simulink model "EJ_01_c"  (R2018a)
settings: Solver=ode23t  StartTime=0.0  StopTime=7  FixedStep=0.01  MaxStep=0.05  RelTol=1e-3  EnableMultiTasking=on
PreLoadFcn:
  | mdl_puma560
values from neighbouring files (symbols this model uses):
  messi = RobotInit(pert)    [Ej_01.m]
  q0 = [0 -pi/2]    [Ej_01.m]
undefined symbols (not defined in the file or in its folder): slcoulomb
libraries: roblocks x6, simulink x1
settings Model: ExtModeTrigMode=oneshot  ExtModeArmWhenConnect=off  Creator=pic  LastModifiedBy=sebas
settings SolverCC: ZeroCrossControl=DisableAll
settings DataIOCC: SaveFormat=Array  SignalLoggingSaveFormat=ModelDataLogs  ReturnWorkspaceOutputs=on  TimeSaveName=t  OutputSaveName=y  ReturnWorkspaceOutputsName=ctorque
settings OptimizationCC: BlockReduction=off  BooleanDataType=off  ExpressionDepthLimit=2147483647  InitFltsAndDblsToZero=on  LifeSpan=inf
settings DebuggingCC: SaveWithParameterizedLinksMsg=none  UnderspecifiedInitializationDetection=Classic  MergeDetectMultiDrivingBlocksExec=none  SignalResolutionControl=TryResolveAllWithWarning  MultiTaskDSMMsg=warning  MultiTaskCondExecSysMsg=none  FcnCallInpInsideContextMsg=warning  AllowSymbolicDim=off  StateNameClashWarn=warning  SFUnexpectedBacktrackingDiag=warning  SFNoUnconditionalDefaultTransitionDiag=warning  SFExecutionAtInitializationDiag=none
settings HardwareCC: ProdBitPerPointer=32  ProdBitPerSizeT=32  ProdBitPerPtrDiffT=32  ProdLargestAtomicFloat=None  ProdIntDivRoundTo=Undefined  ProdEndianess=Unspecified  ProdWordSize=32  ProdHWDeviceType=32-bit Generic  TargetUnknown=on
settings ModelReferenceCC: PropagateSignalLabelsOutOfModel=off
settings CodeAppCC: StateflowObjectComments=on
settings GRTTargetCC: TargetLangStandard=C89/C90 (ANSI)  ModelReferenceCompliant=off  CompOptLevelCompliant=off  GeneratePreprocessorConditionals=Disable all  CombineOutputUpdateFcns=off  MatFileLogging=off  GRTInterface=on
settings ConfigComp: CovMetricSettings=dw  CovHtmlReporting=on  CovSaveCumulativeToWorkspaceVar=on  CovSaveSingleToWorkspaceVar=on  CovExternalEMLEnable=off

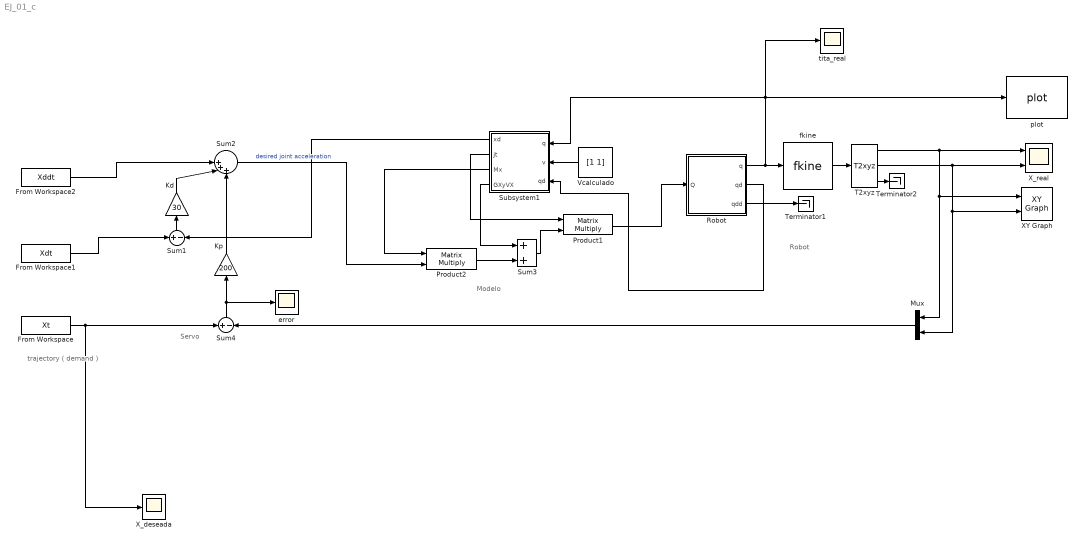
== system EJ_01_c ==
  note: Modelo
  note: trajectory
      | ( demand )
  note: Servo
  note: Robot
  From Workspace : FromWorkspace  VariableName=Xt  OutputAfterFinalValue=Holding final value
  From Workspace1 : FromWorkspace  VariableName=Xdt  OutputAfterFinalValue=Holding final value
  From Workspace2 : FromWorkspace  VariableName=Xddt  OutputAfterFinalValue=Holding final value
  Kd : Gain  Gain=30  SaturateOnIntegerOverflow=on  OutDataTypeStr=Inherit: Same as input  ParamDataTypeStr=Inherit: Same as input
  Kp : Gain  Gain=200  SaturateOnIntegerOverflow=on  OutDataTypeStr=Inherit: Same as input  ParamDataTypeStr=Inherit: Same as input
  Mux : Mux  Inputs=2
  Product1 : Product  Multiplication=Matrix(*)
  Product2 : Product  Multiplication=Matrix(*)
  Robot : Subsystem  AncestorBlock=roblocks/Arm/Robot  mask{robot=messi, q0=q0}
      mask prompts: robot "Robot object"; q0 "Initial state"
      mask help: Rigid-body dynamic model of robot.
      mask init:
      | if isa(robot, 'SerialLink')
      |     rname = robot.name;
      |     %fprintf('**robot name is %s\n', rname);
      | else
      |     rname = '';
      |     n = 0
      | end
      mask Help:
      | Simulates the forward (direct) rigid-body dynamics of the robot described
      | by the given robot object.  For given applied joint torque/force it computes
      | the instaneous joint coordinates, velocities and acclerations.
      | 
      | 
      | <b>Parameters::</b>
      | 
      | robot (SerialLink) a dynamic model of an N-link serial link manipulator
      | q0 (1xN)  Initial joint coordinates
      | 
      | <b>Inputs::</b>
      | 
      | Q (1xN) the generalized joint force (torque or force) required to achieve
      | the motion state (q, qd, qdd).
      | 
      | <b>Outputs::</b>
      | 
      | q (1xN) joint coordinates
      | qd (1xN) joint coordinate velocity
      | qdd (1xN) joint coordinate acceleration
      | 
      | 
      | <b>Notes::</b>
      | 
      | - Required to simulate robot rigid body motion.
      | - Implemented using the recursive Newton-Euler scheme (RNE).
      | - A wrapper for the Toolbox method accel() which in turn depends on the
      |   method rne().
      mask Display:
      | port_label('input', 1, 'Q')
      | port_label('output', 1, 'q')
      | port_label('output', 2, 'qd')
      | port_label('output', 3, 'qdd')
      | text(0.1, 0.9,  rname, 'horizontalAlignment', 'left')
  Subsystem1 : Subsystem
  Sum1 : Sum  Inputs=+|-  SaturateOnIntegerOverflow=on  InputSameDT=on  OutDataTypeStr=Inherit: Same as first input
  Sum2 : Sum  Inputs=||+++  SaturateOnIntegerOverflow=on  InputSameDT=on  OutDataTypeStr=Inherit: Same as first input
  Sum3 : Sum
  Sum4 : Sum  Inputs=+|-  SaturateOnIntegerOverflow=on  InputSameDT=on  OutDataTypeStr=Inherit: Same as first input
  T2xyz : roblocks/Toolbox/T2xyz
  Terminator1 : Terminator
  Terminator2 : Terminator
  Vcalculado : Constant  Value=[1 1]
  XY Graph : simulink/Sinks/XY Graph  xmin=0  xmax=2  ymin=-1.5  ymax=2  st=-1
  X_deseada : Scope
  X_real : Scope  NumInputPorts=2
  error : Scope
  fkine : roblocks/Arm/fkine  robot=messi
  plot : roblocks/Arm/plot  robot=messi  fps=10  holdplot=on
  tita_real : Scope
  wires:
  Robot/3(qdd) -> Terminator1/1
  fkine/1 -> T2xyz/1
  T2xyz/2 -> Mux/2, XY Graph/2, X_real/2
  T2xyz/1 -> Mux/1, XY Graph/1, X_real/1
  Sum1/1 -> Kd/1
  Sum4/1 -> Kp/1, error/1
  From Workspace/1 -> Sum4/1, X_deseada/1
  From Workspace1/1 -> Sum1/1
  Kp/1 -> Sum2/3
  Kd/1 -> Sum2/2
  From Workspace2/1 -> Sum2/1
  Mux/1 -> Sum4/2
  Robot/1(q) -> tita_real/1, Subsystem1/1(q), plot/1, fkine/1
  Robot/2(qd) -> Subsystem1/3(qd)
  T2xyz/3 -> Terminator2/1
  Vcalculado/1 -> Subsystem1/2(v)
  Product1/1 -> Robot/1(Q)
  Subsystem1/1("xd ") -> Sum1/2
  Subsystem1/3(Mx) -> Product2/1
  Sum2/1 -> Product2/2  "desired joint acceleration"
  Subsystem1/2(jt) -> Product1/1
  Sum3/1 -> Product1/2
  Subsystem1/4(GXyVX) -> Sum3/1
  Product2/1 -> Sum3/2

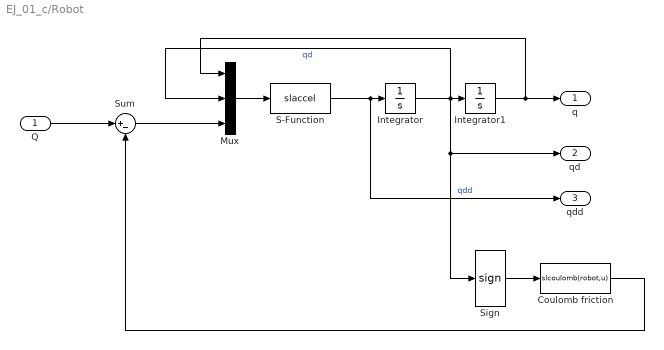
== system EJ_01_c/Robot ==
  Q : Inport
  Coulomb friction : MATLABFcn  MATLABFcn=slcoulomb(robot,u)  OutputDimensions=[robot.n 1]  Output1D=off
  Integrator : Integrator
  Integrator1 : Integrator  InitialCondition=q0
  Mux : Mux  Inputs=3
  S-Function : S-Function  FunctionName=slaccel  Parameters=robot  SFunctionDeploymentMode=off  EnableBusSupport=off
  Sign : Signum
  Sum : Sum  Inputs=|+-
  q : Outport
  qd : Outport  Port=2
  qdd : Outport  Port=3
  wires:
  S-Function/1 -> qdd/1, Integrator/1  "qdd"
  Mux/1 -> S-Function/1
  Integrator/1 -> Sign/1, qd/1, Integrator1/1, Mux/2  "qd"
  Integrator1/1 -> q/1, Mux/1
  Q/1 -> Sum/1
  Sum/1 -> Mux/3
  Coulomb friction/1 -> Sum/2
  Sign/1 -> Coulomb friction/1

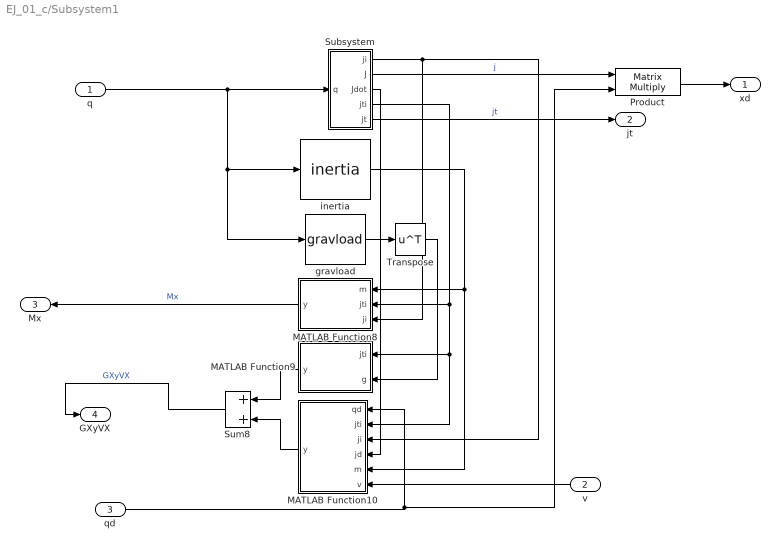
== system EJ_01_c/Subsystem1 ==
  q : Inport
  v : Inport  Port=2
  qd : Inport  Port=3
  MATLAB Function10 : MATLAB Function  TreatAsAtomicUnit=on
  MATLAB Function8 : MATLAB Function  TreatAsAtomicUnit=on
  MATLAB Function9 : MATLAB Function  TreatAsAtomicUnit=on
  Product : Product  Multiplication=Matrix(*)
  Subsystem : Subsystem
  Sum8 : Sum
  Transpose : Math  Operator=transpose  SaturateOnIntegerOverflow=on
  gravload : roblocks/Arm/gravload  robot=messi
  inertia : roblocks/Arm/inertia  robot=messi
  "xd " : Outport  VectorParamsAs1DForOutWhenUnconnected=on
  jt : Outport  Port=2  VectorParamsAs1DForOutWhenUnconnected=on
  Mx : Outport  Port=3  VectorParamsAs1DForOutWhenUnconnected=on
  GXyVX : Outport  Port=4  VectorParamsAs1DForOutWhenUnconnected=on
  wires:
  Subsystem/1(ji) -> MATLAB Function8/3(ji), MATLAB Function10/3(ji)
  q/1 -> gravload/1, inertia/1, Subsystem/1(q)
  Subsystem/4(jti) -> MATLAB Function8/2(jti), MATLAB Function9/1(jti), MATLAB Function10/2(jti)
  MATLAB Function9/1(y) -> Sum8/1
  Sum8/1 -> GXyVX/1  "GXyVX"
  Subsystem/3(Jdot) -> MATLAB Function10/4(jd)
  MATLAB Function10/1(y) -> Sum8/2
  inertia/1 -> MATLAB Function8/1(m), MATLAB Function10/5(m)
  Subsystem/5(jt) -> jt/1  "jt"
  v/1 -> MATLAB Function10/6(v)
  qd/1 -> Product/2, MATLAB Function10/1(qd)
  MATLAB Function8/1(y) -> Mx/1  "Mx"
  gravload/1 -> Transpose/1
  Transpose/1 -> MATLAB Function9/2(g)
  Subsystem/2(J) -> Product/1  "j"
  Product/1 -> "xd "/1

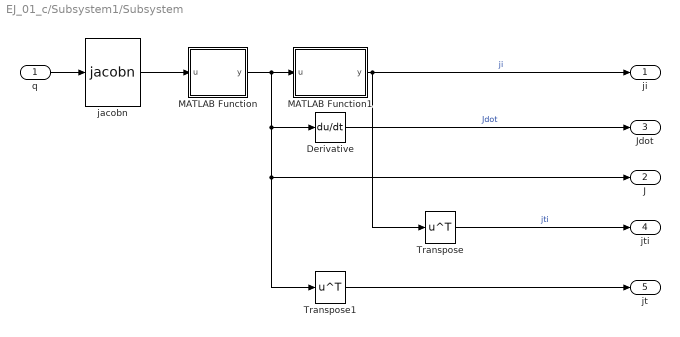
== system EJ_01_c/Subsystem1/Subsystem ==
  q : Inport
  Derivative : Derivative
  MATLAB Function : MATLAB Function  TreatAsAtomicUnit=on
  MATLAB Function1 : MATLAB Function  TreatAsAtomicUnit=on
  Transpose : Math  Operator=transpose  SaturateOnIntegerOverflow=on
  Transpose1 : Math  Operator=transpose  SaturateOnIntegerOverflow=on
  jacobn : roblocks/Arm/jacobn  robot=messi
  ji : Outport  VectorParamsAs1DForOutWhenUnconnected=on
  J : Outport  Port=2  VectorParamsAs1DForOutWhenUnconnected=on
  Jdot : Outport  Port=3  VectorParamsAs1DForOutWhenUnconnected=on
  jti : Outport  Port=4  VectorParamsAs1DForOutWhenUnconnected=on
  jt : Outport  Port=5  VectorParamsAs1DForOutWhenUnconnected=on
  wires:
  MATLAB Function1/1(y) -> Transpose/1, ji/1  "ji"
  Transpose/1 -> jti/1  "jti"
  q/1 -> jacobn/1
  Derivative/1 -> Jdot/1  "Jdot"
  Transpose1/1 -> jt/1
  jacobn/1 -> MATLAB Function/1(u)
  MATLAB Function/1(y) -> MATLAB Function1/1(u), J/1, Transpose1/1, Derivative/1

== matlab function EJ_01_c/Subsystem1/Subsystem/MATLAB Function1 ==
  data: u input; y output
function y = inversJac(u)

y = u^(-1);

== matlab function EJ_01_c/Subsystem1/Subsystem/MATLAB Function ==
  data: u input; y output
function y = extract(u)

y = u(1:2,1:2);

== matlab function EJ_01_c/Subsystem1/MATLAB Function8 ==
  data: m input; y output; jti input; ji input
function y = Mx(m,jti,ji)

y = jti*m*ji;

== matlab function EJ_01_c/Subsystem1/MATLAB Function9 ==
  data: jti input; y output; g input
function y = Gx(jti,g)

y = jti*g;

== matlab function EJ_01_c/Subsystem1/MATLAB Function10 ==
  data: qd input; y output; jti input; ji input; jd input; m input; v input
function y = Vx(qd,jti,ji,jd,m,v)

y = jti*(v-m*ji*jd*qd);
